simulink model "computed_torque"  (R2022b)
settings: Solver=VariableStepAuto  StartTime=0.0  StopTime=30.0  RelTol=1e-3
undefined symbols (not defined in the file or in its folder): Lamda, sigbuilder_block
settings Model: Creator=alexi  LastModifiedBy=alexi

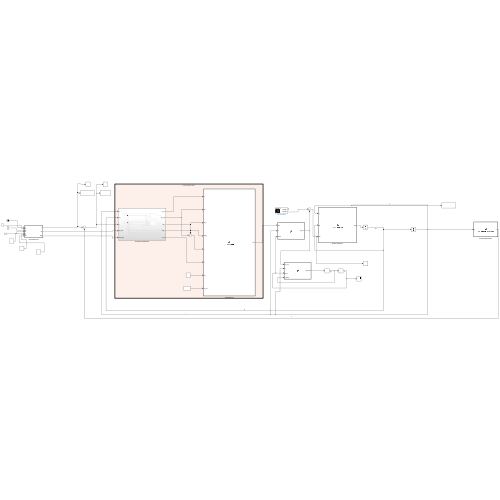
[thumbnail: Simulink's stored preview of the top-level diagram]
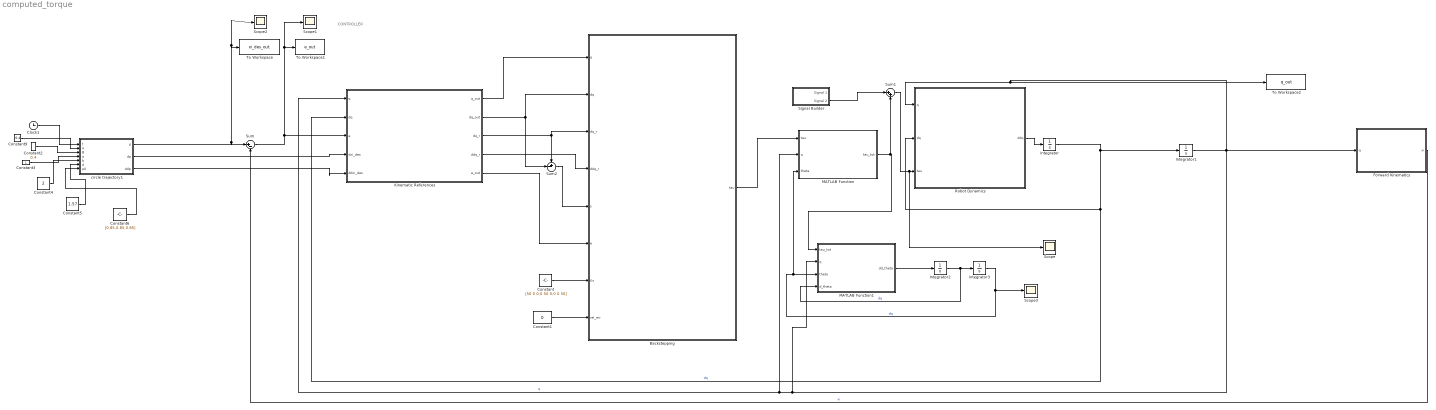
== system computed_torque ==
  note: CONTROLLER
  Backstepping : MATLAB Function  TreatAsAtomicUnit=on
  Clock1 : Clock
  Constant : Constant  Value=[50 0 0;0 50 0;0 0 50]
  Constant1 : Constant  Value=0
  Constant2 : Constant  Value=0.4
  Constant3 : Constant
  Constant4 : Constant  Value=2
  Constant5 : Constant  Value=1.57
  Constant6 : Constant  Value=[0.85,0.85,0.85]
  Constant9 : Constant  Value=0.4
  Forward Kinematics : MATLAB Function  TreatAsAtomicUnit=on
  Integrator : Integrator  InitialCondition=[0,0,0]'
  Integrator1 : Integrator  InitialCondition=[0.25,0.25,0.25]'
  Integrator2 : Integrator  InitialCondition=[0,0,0,0,0,0]'
  Integrator3 : Integrator  InitialCondition=[0,0,0,0,0,0]'
  Kinematic References : Subsystem
  MATLAB Function : MATLAB Function  TreatAsAtomicUnit=on
  MATLAB Function1 : MATLAB Function  TreatAsAtomicUnit=on
  Robot Dynamics : MATLAB Function  TreatAsAtomicUnit=on
  Scope{,1..3} (4 alike) : Scope
  Signal Builder : Subsystem  Tag=STV Subsys  LoadFcn=sigbuilder_block('load');  StartFcn=sigbuilder_block('start');  StopFcn=sigbuilder_block('stop');  ClipboardFcn=sigbuilder_block('clipboard');  mask(Sigbuilder block){tuvar=[0:10]}
      mask help: Simulink:masks:SigbuilderBlock_MD
      mask init:
      | if ~strcmp(get_param(bdroot(gcbh),'SimulationStatus'),'stopped') tuvar = sigbuilder_block('maskInit'); end
      settings: CopyFcn=sigbuilder_block('copy');  DeleteFcn=sigbuilder_block('delete');  ModelCloseFcn=sigbuilder_block('modelClose');  PreSaveFcn=sigbuilder_block('preSave');  PauseFcn=sigbuilder_block('pause');  ContinueFcn=sigbuilder_block('continue');  NameChangeFcn=sigbuilder_block('namechange');  OpenFcn=sigbuilder_block('open',[5.4 30 1141.2 522.6 ]);  CloseFcn=sigbuilder_block('close');
      mask Display: plot(0, 0, 100, 100,[2, 2, 32, 32, 2], [68, 8, 8, 68, 68],[32, 2], [38, 38], [32, 19, 2],[53, 60, 44], [32, 17, 17, 2],[16, 16, 31, 31]);txt = getActiveGroup(gcbh);text(2, 100, txt,'verticalAlignment', 'top');
  Sum : Sum  Inputs=|+-
  Sum1 : Sum  Inputs=|++
  Sum2 : Sum  Inputs=+-|
  To Workspace : ToWorkspace  VariableName=xi_des_out  SaveFormat=Timeseries  SampleTime=-1
  To Workspace1 : ToWorkspace  VariableName=e_out  SaveFormat=Timeseries  SampleTime=-1
  To Workspace2 : ToWorkspace  VariableName=q_out  SaveFormat=Timeseries  SampleTime=-1
  circle trajectory1 : MATLAB Function  TreatAsAtomicUnit=on
  wires:
  Kinematic References/4(ddq_r) -> Backstepping/4(ddq_r)
  circle trajectory1/1(p) -> Scope2/1, To Workspace/1, Sum/1
  Kinematic References/2(dq_out) -> Sum2/2, Backstepping/2(dq)
  Sum2/1 -> Backstepping/5(s)
  circle trajectory1/3(ddp) -> Kinematic References/5(ddxi_des)
  Constant/1 -> Backstepping/7(Ks)
  Forward Kinematics/1(xi) -> Sum/2  "xi"
  Kinematic References/1("q_out ") -> Backstepping/1(q)
  Integrator/1 -> Robot Dynamics/2(dq), Kinematic References/2(dq), Integrator1/1  "dq"
  Sum/1 -> Kinematic References/3(e), To Workspace1/1, Scope1/1
  Integrator1/1 -> MATLAB Function1/2(q), MATLAB Function/2(q), Kinematic References/1(q), Forward Kinematics/1(q), Robot Dynamics/1(q), To Workspace2/1  "q"
  circle trajectory1/2(dp) -> Kinematic References/4(dxi_des)
  Robot Dynamics/1(ddq) -> Integrator/1
  Kinematic References/3(dq_r) -> Backstepping/3(dq_r), Sum2/1
  Kinematic References/5(e_out) -> Backstepping/6(e)
  Clock1/1 -> circle trajectory1/1(t)
  Constant1/1 -> Backstepping/8(rel_err)
  Constant9/1 -> circle trajectory1/2(A)
  Constant2/1 -> circle trajectory1/3(B)
  Constant3/1 -> circle trajectory1/4(a)
  Constant4/1 -> circle trajectory1/5(b)
  Constant5/1 -> circle trajectory1/6(d)
  Constant6/1 -> circle trajectory1/7(p0)
  Backstepping/1(tau) -> MATLAB Function/1(tau)
  MATLAB Function1/1(dd_theta) -> Integrator2/1
  Integrator2/1 -> MATLAB Function1/4(d_theta), Integrator3/1  "dq"
  MATLAB Function/1(tau_tot) -> MATLAB Function1/1(tau_tot), Sum1/2
  Integrator3/1 -> Scope3/1, MATLAB Function/3(theta), MATLAB Function1/3(theta)  "dq"
  Sum1/1 -> Scope/1, Robot Dynamics/3(tau)
  Signal Builder/2(Signal 2) -> Sum1/1

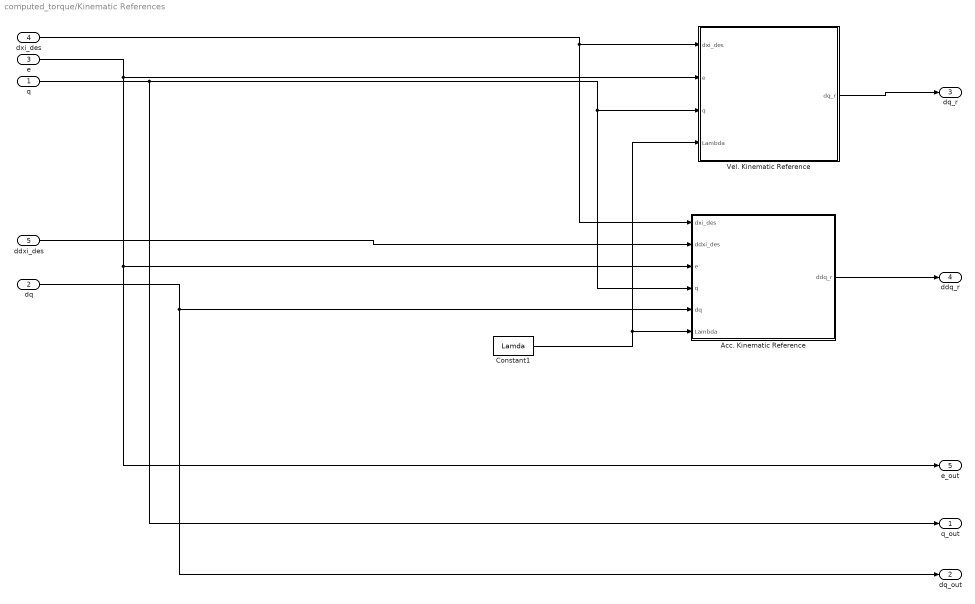
== system computed_torque/Kinematic References ==
  q : Inport
  dq : Inport  Port=2
  e : Inport  Port=3
  dxi_des : Inport  Port=4
  ddxi_des : Inport  Port=5
  Acc. Kinematic Reference : MATLAB Function  TreatAsAtomicUnit=on
  Constant1 : Constant  Value=Lamda
  "Vel. Kinematic Reference " : MATLAB Function  TreatAsAtomicUnit=on
  "q_out " : Outport  VectorParamsAs1DForOutWhenUnconnected=off
  dq_out : Outport  Port=2  VectorParamsAs1DForOutWhenUnconnected=off
  dq_r : Outport  Port=3  VectorParamsAs1DForOutWhenUnconnected=off
  ddq_r : Outport  Port=4  VectorParamsAs1DForOutWhenUnconnected=off
  e_out : Outport  Port=5  VectorParamsAs1DForOutWhenUnconnected=off
  wires:
  ddxi_des/1 -> Acc. Kinematic Reference/2(ddxi_des)
  e/1 -> e_out/1, Acc. Kinematic Reference/3(e), "Vel. Kinematic Reference "/2(e)
  dxi_des/1 -> Acc. Kinematic Reference/1(dxi_des), "Vel. Kinematic Reference "/1(dxi_des)
  Constant1/1 -> "Vel. Kinematic Reference "/4(Lambda), Acc. Kinematic Reference/6(Lambda)
  "Vel. Kinematic Reference "/1(dq_r) -> dq_r/1
  dq/1 -> dq_out/1, Acc. Kinematic Reference/5(dq)
  q/1 -> "q_out "/1, Acc. Kinematic Reference/4(q), "Vel. Kinematic Reference "/3(q)
  Acc. Kinematic Reference/1(ddq_r) -> ddq_r/1

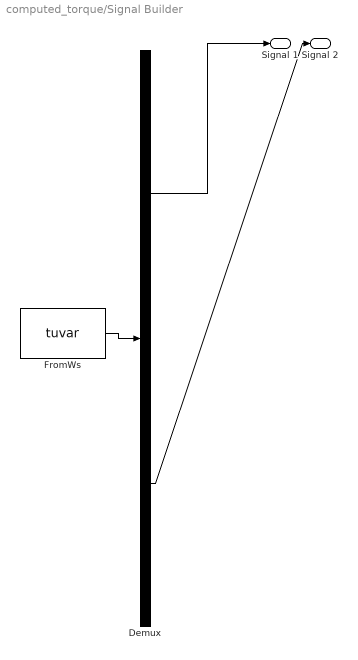
== system computed_torque/Signal Builder ==
  Demux : Demux  Tag=STV Demux  Outputs=2
      settings: DisplayOption=none
  FromWs : FromWorkspace  Tag=STV FromWs  VariableName=tuvar
      SigBuilderData=|
      | common.afterFinalStr = 'Extrapolate'
      | common.sampleTime = 0
      | dataSet.timeRange = [0 10]
      | dataSet.name = 'Group 1'
      | sbobj.Groups.Name = 'Group 1'
      | sbobj.Groups.Signals(1).Name = 'Signal 1'
      | sbobj.Groups.Signals(1).XData = [0 4 4 5.9 5.9 10]
      | sbobj.Groups.Signals(1).YData = [0 0 15.1 15.1 0 0]
      | sbobj.Groups.Signals(2).Name = 'Signal 2'
      | sbobj.Groups.Signals(2).XData = [0 10]
      | sbobj.Groups.Signals(2).YData = [0 0]
  Signal 1 : Outport  Tag=STV Outport
  Signal 2 : Outport  Tag=STV Outport  Port=2
  wires:
  FromWs/1 -> Demux/1
  Demux/1 -> Signal 1/1
  Demux/2 -> Signal 2/1

== matlab function computed_torque/Kinematic References/Acc. Kinematic Reference ==
  data: dxi_des input; ddq_r output; ddxi_des input; e input; q input; dq input; Lambda input
function ddq_r = acc_kinematic_reference(dxi_des, ddxi_des, e, q, dq, Lambda)

coder.extrinsic('disp');

J = zeros(3,3);
dJ = zeros(3,3);

dq1 = dq(1);
dq2 = dq(2);
dq3 = dq(3);

q1 = q(1);
q2 = q(2);
q3 = q(3);

a1 = 1;
a2 = 1;
a3 = 1;

% Computing jacobian and derivative
J = [- a1*sin(q1) - a3*cos(q3)*(cos(q1)*sin(q2) + cos(q2)*sin(q1)) - a2*cos(q1)*sin(q2) - a2*cos(q2)*sin(q1), -a3*cos(q3)*(cos(q1)*sin(q2) +cos(q2)*sin(q1)) - a2*cos(q1)*sin(q2) - a2*cos(q2)*sin(q1), -a3*sin(q3)*(cos(q1)*cos(q2) - sin(q1)*sin(q2)); ...
    a1*cos(q1) + a3*cos(q3)*(cos(q1)*cos(q2) - sin(q1)*sin(q2)) + a2*cos(q1)*cos(q2) - a2*sin(q1)*sin(q2),   a3*cos(q3)*(cos(q1)*cos(q2) - sin(q1)*sin(q2)) + a2*cos(q1)*cos(q2) - a2*sin(q1)*sin(q2),  -a3*sin(q3)*(cos(q1)*sin(q2) + cos(q2)*sin(q1)); ...
    0,0,- a3*cos(q3)*(cos(q1)*sin(q2) + cos(q2)*sin(q1))^2 - a3*cos(q3)*(cos(q1)*cos(q2) - sin(q1)*sin(q2))^2];

a11 = -a1*dq1*cos(q1)-a3*(dq1*cos(q1+q2)+ dq2*cos(q1+q2))*sin(q3)-a2*(dq1*cos(q1+q2)+ dq2*cos(q1+q2));
a12 = -a3*( dq1*cos(q1+q2)+ dq2*cos(q1+q2))*sin(q3)-a2*( dq1*cos(q1+q2)+ dq2*cos(q1+q2));
a13 = -a3*( dq1*cos(q1+q2)+ dq2*cos(q1+q2))*cos(q3);
a21 = -a1*dq1*sin(q1)-a3*( dq1*sin(q1+q2)+ dq2*sin(q1+q2))*cos(q3)-a2*( dq1*sin(q1+q2)+ dq2*sin(q1+q2));
a22 = -a3*(dq1*sin(q1+q2)+dq2*sin(q1+q2))*sin(q3)-a2*(dq1*sin(q1+q2)+dq2*sin(q1+q2));
a23 = -a3*(dq1*cos(q1+q2)+dq2*cos(q1+q2))*sin(q3);
a31 = 0;
a32 = 0;
a33 = 2*a3*(dq1*cos(q1+q2)+dq2*cos(q1+q2))*sin(q1+q2)*sin(q3)-2*a3*(dq1*sin(q1+q2)+dq2*sin(q1+q2))*cos(q1+q2)*sin(q3);

dJ = [a11,a12,a13;a21,a22,a23;a31,a32,a33];

ddq_r = inv(J) * (ddxi_des + Lambda*dxi_des - Lambda*J*dq) ...
- inv(J)*dJ*inv(J)*(dxi_des + Lambda*e);
end

== matlab function computed_torque/circle trajectory1 ==
  data: t input; p output; dp output; ddp output; A input; B input; a input; b input; d input; p0 input
function [p,dp,ddp] = lissajous(t,A,B,a,b,d,p0)
C = 0.1;  % Ampiezza dell'oscillazione in z
c = 0.2;  % Frequenza in z
phi = pi/4;
p = [A*sin(a*t+d); B*sin(b*t);C*sin(c*t + phi)] + p0;
dp = [A*a*cos(a*t+d); B*b*cos(b*t);C*c*cos(c*t+phi)];
ddp = [-A*a^2*sin(a*t+d); -B*b^2*sin(b*t);-C*c^2*sin(c*t+phi)];
% a = 0.2;    % Ampiezza lungo l'asse X
% b = 0.2;    % Ampiezza lungo l'asse Y
% p0 = [1;0.8;0.8];
% 
% x = a * cos(t);
% y = b * sin(t);
% z =  0.1 * sin(t);
% 
% p = [x y z]'+p0;
% 
% dx = -a*sin(t);
% dy = b*cos(t);
% dz = 0.5*cos(t);
% 
% dp = [dx dy dz]';
% 
% ddx = -a*cos(t);
% ddy = -b*sin(t);
% ddz = -0.5*sin(t);
% 
% ddp = [ddx ddy ddz]';

== matlab function computed_torque/Kinematic References/Vel. Kinematic Reference  ==
  data: dxi_des input; dq_r output; e input; q input; Lambda input
function dq_r = vel_kinematic_reference(dxi_des, e, q, Lambda)
a1 = 1;
a2 = 1;
a3 = 1;

q1 = q(1);
q2 = q(2);
q3 = q(3);

% Computing jacobian
J = [- a1*sin(q1) - a3*cos(q3)*(cos(q1)*sin(q2) + cos(q2)*sin(q1)) - a2*cos(q1)*sin(q2) - a2*cos(q2)*sin(q1), -a3*cos(q3)*(cos(q1)*sin(q2) +cos(q2)*sin(q1)) - a2*cos(q1)*sin(q2) - a2*cos(q2)*sin(q1), -a3*sin(q3)*(cos(q1)*cos(q2) - sin(q1)*sin(q2)); ...
    a1*cos(q1) + a3*cos(q3)*(cos(q1)*cos(q2) - sin(q1)*sin(q2)) + a2*cos(q1)*cos(q2) - a2*sin(q1)*sin(q2),   a3*cos(q3)*(cos(q1)*cos(q2) - sin(q1)*sin(q2)) + a2*cos(q1)*cos(q2) - a2*sin(q1)*sin(q2),  -a3*sin(q3)*(cos(q1)*sin(q2) + cos(q2)*sin(q1)); ...
    0,0,- a3*cos(q3)*(cos(q1)*sin(q2) + cos(q2)*sin(q1))^2 - a3*cos(q3)*(cos(q1)*cos(q2) - sin(q1)*sin(q2))^2];

dq_r = inv(J) * (dxi_des + Lambda*e);
end

== matlab function computed_torque/Backstepping ==
  data: q input; dq input; dq_r input; ddq_r input; s input; e input; Ks input; rel_err input; tau output
function tau  = backstepping(q, dq, dq_r, ddq_r, s, e, Ks, rel_err)

coder.extrinsic('disp');

% Get dynamic matrices
B = RRR_mass_matrix(q);
C = RRR_coriolis_matrix(q,dq);
G = RRR_gravity_matrix(q);

% Adding uncertainty
B = B.*(1 + rel_err);
C = C.*(1 + rel_err);
G = G.*(1 + rel_err);

a1 = 1;
a2 = 1;
a3 = 1;
q1 = q(1);
q2 = q(2);
q3 = q(3);
% Get Jacobian
J = [- a1*sin(q1) - a3*cos(q3)*(sin(q1+q2)) - a2*sin(q1+q2), -a3*cos(q3)*(sin(q1+q2)) - a2*sin(q1+q2), -a3*sin(q3)*(cos(q1+q2)); ...
    a1*cos(q1) + a3*cos(q3)*(cos(q1+q2)) + a2*cos(q1+q2),   a3*cos(q3)*(cos(q1+q2)) + a2*cos(q1+q2),  -a3*sin(q3)*(sin(q1+q2)); ...
    0,0,- a3*cos(q3)*(sin(q1+q2))^2 - a3*cos(q3)*(cos(q1+q2))^2];

% Control law
tau = B*ddq_r + C*dq_r + G + Ks*s + J.'*e;

== matlab function computed_torque/Robot Dynamics ==
  data: q input; dq input; tau input; ddq output
function ddq = inverse_dynamics(q, dq, tau)

% Get dynamic matrices
B = RRR_mass_matrix(q);
C = RRR_coriolis_matrix(q,dq);
G = RRR_gravity_matrix(q);
ddq = pinv(B)*(tau - C*dq - G);

== matlab function computed_torque/Forward Kinematics ==
  data: q input; xi output
function xi  = RR_forward_kinematics(q)

    q1 = q(1);
    q2 = q(2);
    q3 = q(3);

    a1 = 1;
    a2 = 1;
    a3 = 1;

    p0 = [0;0;0];
    p1 = [a1*cos(q1); a1*sin(q1);0];
    p2 = p1+[a2*cos(q1+q2);a2*sin(a1+q2);0];
    xi = [a1*cos(q1) + a3*cos(q3)*(cos(q1)*cos(q2) - sin(q1)*sin(q2)) + a2*cos(q1)*cos(q2) - a2*sin(q1)*sin(q2); a1*sin(q1) + a3*cos(q3)*(cos(q1)*sin(q2) + cos(q2)*sin(q1)) + a2*cos(q1)*sin(q2) + a2*cos(q2)*sin(q1);-a3*sin(q3)];
end

== matlab function computed_torque/MATLAB Function ==
  data: tau input; tau_tot output; q input; theta input
function tau_tot  = fcn(tau,q,theta)
K1 = 0.5;
K2 = 0.5;
q1 = q(1);
q2 = q(2);
q3 = q(3);
theta1_q1 = theta(1);
theta2_q1 = theta(2);
theta1_q2 = theta(3);
theta2_q2 = theta(4);
theta1_q3 = theta(5);
theta2_q3 = theta(6);

tau_e_q1 = K1*(q1-theta1_q1)+K2*(q1-theta2_q1);
tau_e_q2 = K1*(q2-theta1_q2)+K2*(q2-theta2_q2);
tau_e_q3 = K1*(q3-theta1_q3)+K2*(q3-theta2_q3);

tau_e_q = [tau_e_q1;tau_e_q2;tau_e_q3];
tau_tot = tau + tau_e_q;

== matlab function computed_torque/MATLAB Function1 ==
  data: tau_tot input; dd_theta output; q input; theta input; d_theta input
function dd_theta  = fcn(tau_tot,q,theta,d_theta)
q1 = q(1);
q2 = q(2);
q3 = q(3);

m1 = 1;
m2 = 1;
m3 = 1;

a1 = 1;
a2 = 1;
a3 = 1;

J1_q1 = 1/24*m1*a1^2;
J2_q1 = 1/24*m1*a1^2;
J1_q2 = 1/24*m2*a2^2;
J2_q2 = 1/24*m2*a2^2;
J1_q3 = 1/24*m3*a3^2;
J2_q3 = 1/24*m3*a3^2;

D1 = 0.1;
D2 = 0.1;

K1 = 20;
K2 = 20;

tau_tot_1 = tau_tot(1);
tau_tot_2 = tau_tot(2);
tau_tot_3 = tau_tot(3);

tau_tot_1_theta1 = tau_tot_1/2;
tau_tot_1_theta2 = tau_tot_1_theta1;

tau_tot_2_theta1 = tau_tot_2/2;
tau_tot_2_theta2 = tau_tot_2_theta1;

tau_tot_3_theta1 = tau_tot_3/2;
tau_tot_3_theta2 = tau_tot_3_theta1;

theta1_q1 = theta(1);
theta2_q1 = theta(2);
theta1_q2 = theta(3);
theta2_q2 = theta(4);
theta1_q3 = theta(5);
theta2_q3 = theta(6);

d_theta1_q1 = d_theta(1);
d_theta2_q1 = d_theta(2);
d_theta1_q2 = d_theta(3);
d_theta2_q2 = d_theta(4);
d_theta1_q3 = d_theta(5);
d_theta2_q3 = d_theta(6);

dd_theta1_q1 = pinv(J1_q1)*(tau_tot_1_theta1+K1*(q1-theta1_q1)-D1*d_theta1_q1);
dd_theta2_q1 = pinv(J2_q1)*(tau_tot_1_theta2+K2*(q1-theta2_q1)-D2*d_theta2_q1);

dd_theta1_q2 = pinv(J1_q2)*(tau_tot_2_theta1+K1*(q2-theta1_q2)-D1*d_theta1_q2);
dd_theta2_q2 = pinv(J2_q2)*(tau_tot_2_theta2+K2*(q2-theta2_q2)-D2*d_theta2_q2);

dd_theta1_q3 = pinv(J1_q3)*(tau_tot_3_theta1+K1*(q3-theta1_q3)-D1*d_theta1_q3);
dd_theta2_q3 = pinv(J2_q3)*(tau_tot_3_theta2+K2*(q3-theta2_q3)-D2*d_theta2_q3);

dd_theta = [dd_theta1_q1;dd_theta2_q1;dd_theta1_q2;dd_theta2_q2;dd_theta1_q3;dd_theta2_q3];
